simulink model "network_armax"  (R2024a)
settings: Solver=FixedStepDiscrete  StartTime=0.0  StopTime=499  FixedStep=1  RelTol=1e-3
values from neighbouring files (symbols this model uses):
  theta = [A1(2:3)' B1' C1(2:3)' A2(2:3)' B2' C2(2:3)' A3(2:3)' B3' C3(2:3)']    [a_generate_100_systems.m]    (also in b_gen_data.m = thetas(i,:); c_gen_100_realizations_system1.m = thetas(1,:))
settings Model: Creator=jogal  LastModifiedBy=jogal
settings OptimizationCC: ReuseModelBlockBuffer=off
settings RTWCC: GPUComputeCapability=3.5

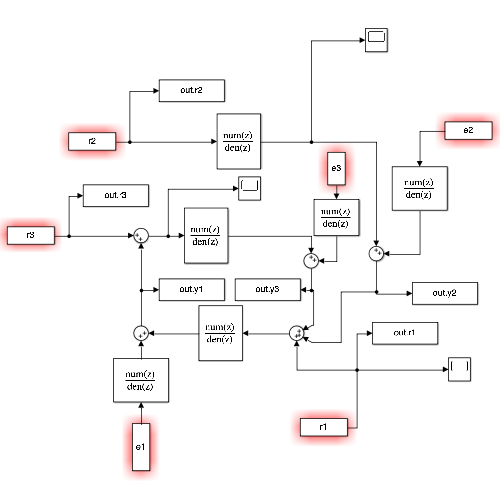
[thumbnail: Simulink's stored preview of the top-level diagram]
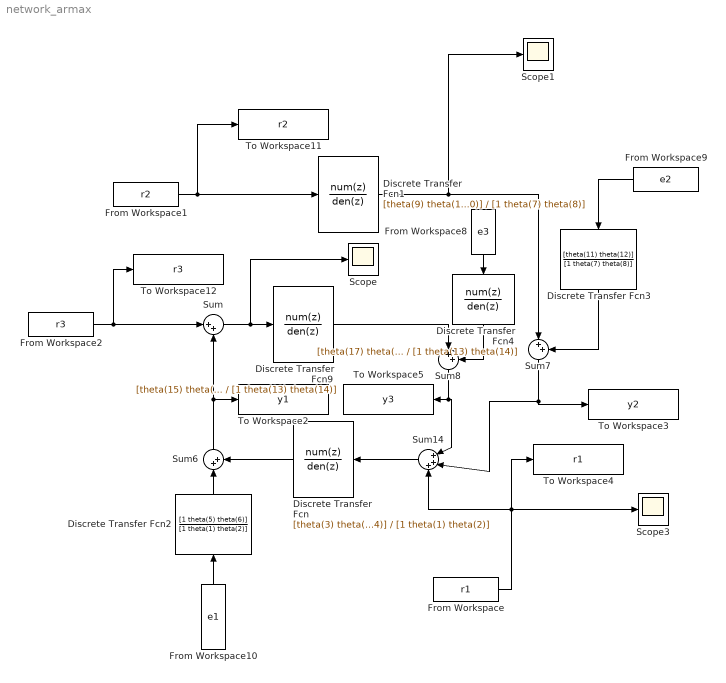
== system network_armax ==
  Discrete Transfer Fcn : DiscreteTransferFcn  Numerator=[theta(3) theta(4)]  Denominator=[1 theta(1) theta(2)]
  Discrete Transfer Fcn1 : DiscreteTransferFcn  Numerator=[theta(9) theta(10)]  Denominator=[1 theta(7) theta(8)]
  Discrete Transfer Fcn2 : DiscreteTransferFcn  Numerator=[1 theta(5) theta(6)]  Denominator=[1 theta(1) theta(2)]
  Discrete Transfer Fcn3 : DiscreteTransferFcn  Numerator=[theta(11) theta(12)]  Denominator=[1 theta(7) theta(8)]
  Discrete Transfer Fcn4 : DiscreteTransferFcn  Numerator=[theta(17) theta(18)]  Denominator=[1 theta(13) theta(14)]
  Discrete Transfer Fcn9 : DiscreteTransferFcn  Numerator=[theta(15) theta(16)]  Denominator=[1 theta(13) theta(14)]
  From Workspace : FromWorkspace  VariableName=r1  SampleTime=1  Interpolate=off  OutputAfterFinalValue=Holding final value
  From Workspace1 : FromWorkspace  VariableName=r2  SampleTime=1  Interpolate=off  OutputAfterFinalValue=Holding final value
  From Workspace10 : FromWorkspace  VariableName=e1  SampleTime=1  Interpolate=off  OutputAfterFinalValue=Holding final value
  From Workspace2 : FromWorkspace  VariableName=r3  SampleTime=1  Interpolate=off  OutputAfterFinalValue=Holding final value
  From Workspace8 : FromWorkspace  VariableName=e3  SampleTime=1  Interpolate=off  OutputAfterFinalValue=Holding final value
  From Workspace9 : FromWorkspace  VariableName=e2  SampleTime=1  Interpolate=off  OutputAfterFinalValue=Holding final value
  Scope : Scope
  Scope1 : Scope
  Scope3 : Scope
  Sum{,6..8} (4 alike) : Sum  Inputs=|++
  Sum14 : Sum  Inputs=|+++
  To Workspace11 : ToWorkspace  VariableName=r2  SampleTime=-1
  To Workspace12 : ToWorkspace  VariableName=r3  SampleTime=-1
  To Workspace2 : ToWorkspace  VariableName=y1  SampleTime=-1
  To Workspace3 : ToWorkspace  VariableName=y2  SampleTime=-1
  To Workspace4 : ToWorkspace  VariableName=r1  SampleTime=-1
  To Workspace5 : ToWorkspace  VariableName=y3  SampleTime=-1
  wires:
  From Workspace1/1 -> To Workspace11/1, Discrete Transfer Fcn1/1
  From Workspace2/1 -> Sum/1, To Workspace12/1
  Sum14/1 -> Discrete Transfer Fcn/1
  Discrete Transfer Fcn/1 -> Sum6/2
  Sum6/1 -> Sum/2, To Workspace2/1
  Sum/1 -> Scope/1, Discrete Transfer Fcn9/1
  Discrete Transfer Fcn9/1 -> Sum8/1
  Sum8/1 -> Sum14/1, To Workspace5/1
  Discrete Transfer Fcn1/1 -> Scope1/1, Sum7/1
  Sum7/1 -> To Workspace3/1, Sum14/2
  From Workspace/1 -> Scope3/1, Sum14/3, To Workspace4/1
  Discrete Transfer Fcn2/1 -> Sum6/1
  From Workspace10/1 -> Discrete Transfer Fcn2/1
  From Workspace9/1 -> Discrete Transfer Fcn3/1
  Discrete Transfer Fcn3/1 -> Sum7/2
  From Workspace8/1 -> Discrete Transfer Fcn4/1
  Discrete Transfer Fcn4/1 -> Sum8/2
